simulink model "mpc_tracking_state"  (R2020b)
settings: Solver=ode4  StartTime=0.0  StopTime=t_sim  FixedStep=T  RelTol=1e-3
values from neighbouring files (symbols this model uses):
  mpc = mpc_design(mpc_param)    [main.m]
  ref = [10; 6; 0; 0]    [main.m]
  T = 0.01    [main.m]
  x0 = [0; 0; 0; 0]    [main.m]
settings Model: Creator=vince  LastModifiedBy=vince
settings DataIOCC: ReturnWorkspaceOutputs=off

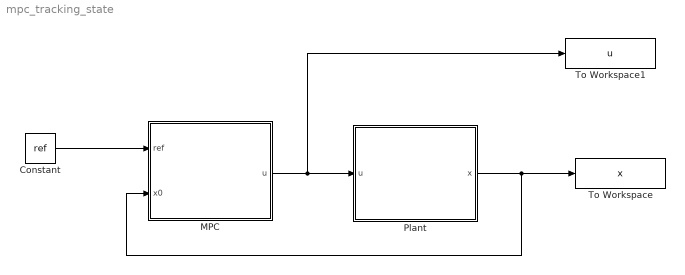
== system mpc_tracking_state ==
  Constant : Constant  Value=ref  SampleTime=-1
  MPC : Subsystem
  Plant : Subsystem
  To Workspace : ToWorkspace  VariableName=x  SaveFormat=Timeseries  SampleTime=-1
  To Workspace1 : ToWorkspace  VariableName=u  SaveFormat=Timeseries  SampleTime=-1
  wires:
  Constant/1 -> MPC/1(ref)
  MPC/1(u) -> To Workspace1/1, Plant/1(u)
  Plant/1(x) -> MPC/2(x0), To Workspace/1

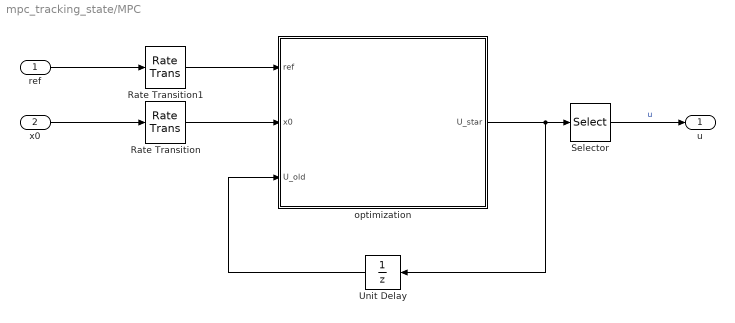
== system mpc_tracking_state/MPC ==
  ref : Inport
  x0 : Inport  Port=2
  Rate Transition : RateTransition  OutPortSampleTime=mpc.Ts
  Rate Transition1 : RateTransition  OutPortSampleTime=mpc.Ts
  Selector : Selector  InputPortWidth=mpc.q*mpc.Nc  IndexOptions=Index vector (dialog)  Indices=1:mpc.q  OutputSizes=1
  Unit Delay : UnitDelay  InitialCondition=mpc.U0  SampleTime=mpc.Ts  HasFrameUpgradeWarning=on
  optimization : MATLAB Function  TreatAsAtomicUnit=on
  u : Outport
  wires:
  optimization/1(U_star) -> Unit Delay/1, Selector/1
  x0/1 -> Rate Transition/1
  Rate Transition1/1 -> optimization/1(ref)
  ref/1 -> Rate Transition1/1
  Rate Transition/1 -> optimization/2(x0)
  Unit Delay/1 -> optimization/3(U_old)
  Selector/1 -> u/1  "u"

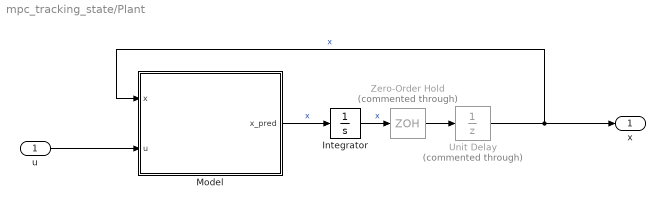
== system mpc_tracking_state/Plant ==
  u : Inport
  Integrator : Integrator  InitialCondition=x0
  Model : MATLAB Function  TreatAsAtomicUnit=on
  Unit Delay : UnitDelay  Commented=through  InitialCondition=x0  SampleTime=T  HasFrameUpgradeWarning=on
  Zero-Order Hold : ZeroOrderHold  Commented=through  SampleTime=T
  x : Outport
  wires:
  Unit Delay/1 -> Model/1(x), x/1  "x"
  u/1 -> Model/2(u)
  Model/1(x_pred) -> Integrator/1  "x"
  Integrator/1 -> Zero-Order Hold/1  "x"
  Zero-Order Hold/1 -> Unit Delay/1

== matlab function mpc_tracking_state/MPC/optimization ==
  data: ref input; U_star output; x0 input; U_old input; mpc parameter
function U_star   = mpc_optimization(ref, x0, U_old, mpc)
%% Documentation
%{
    IN: ref, x, U_old
    OUT: U*
%}


%% Reference
REF = repmat(ref, mpc.Np, 1);



%% Constraints
X_min = mpc.X_c(:,1);
X_max = mpc.X_c(:,2);
U_min = mpc.U_c(:,1);
U_max = mpc.U_c(:,2);
dU_min = mpc.dU_c(:,1);
dU_max = mpc.dU_c(:,2);

A_ineq = [-mpc.B_bar; 
          mpc.B_bar;
          -eye(mpc.q*mpc.Nc); 
          eye(mpc.q*mpc.Nc); 
          -eye(mpc.q*mpc.Nc); 
          eye(mpc.q*mpc.Nc)];
b_ineq = [-X_min+mpc.A_bar*x0; 
          X_max-mpc.A_bar*x0;
          -U_min; 
          U_max;
          -dU_min-U_old; 
          dU_max+U_old];



%% Objective function
H = mpc.R_bar + mpc.B_bar'*mpc.Q_bar*mpc.B_bar;
H = (H+H')/2;
f = (mpc.A_bar*x0-REF)'*mpc.Q_bar*(mpc.B_bar);



%% Optimization: J(u(k)) = U(k)'*H*U(k) + f'*U(k)
coder.extrinsic('quadprog');
% options = optimoptions('quadprog', 'Algorithm', 'active-set', 'Display', 'iter');

U_star = zeros(mpc.q*mpc.Nc, 1);
U_star = quadprog(H, f, A_ineq, b_ineq, [], [], [], [], []);

== matlab function mpc_tracking_state/Plant/Model ==
  data: x input; u input; x_pred output
function x_pred = mpc_pred_disc(x, u)


A = [0 0 1 0; 0 0 0 1; 0 0 0 0; 0 0 0 0];
B = [0 0; 0 0; 1 0; 0 1];
C = [1 0 0 0; 0 1 0 0];
D = zeros(size(C,1), size(B,2));
x0 = x;

x_pred = A*x0 + B*u;
